simulink model "model1a"  (R2014b)
settings: Solver=ode45  StartTime=0.0  StopTime=30.0  RelTol=1e-3
settings Model: Creator=Shane Reynolds  LastModifiedBy=Shane Reynolds

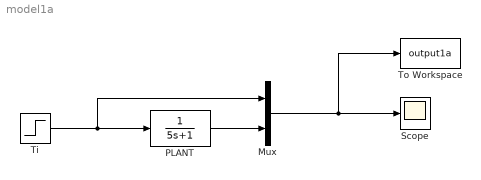
== system model1a ==
  Mux : Mux  Inputs=2
  PLANT : TransferFcn  Denominator=[5 1]
  Scope : Scope
  Ti : Step  After=10  SampleTime=0
  To Workspace : ToWorkspace  VariableName=output1a  SaveFormat=Timeseries  SampleTime=-1
  wires:
  Ti/1 -> Mux/1, PLANT/1
  PLANT/1 -> Mux/2
  Mux/1 -> To Workspace/1, Scope/1
